simulink library "Pipe_Isolation"  (Simulink 8.2)
settings: Solver=ode45  StartTime=0.0  StopTime=10.0  RelTol=1e-3
libraries: carnot x4
settings Model: Creator=lena.frank  LastModifiedBy=drhf

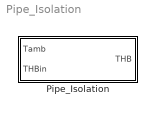
== system Pipe_Isolation ==
  Pipe_Isolation : Subsystem  mask(pipe with relative isolation thickness){dia=0.02, len=10, hgt=0, isolat=43.72, condiso=0.05, cond=0, cwall=1000, t0=20, lin=100/0.2, qua=100/0.2^2, nodes=10}
      mask prompts: dia "Diameter [m]"; len "Length of pipe [m]"; hgt "difference in static height [m], positive for outlet above"; isolat "Isolation thickness in % (100%: isolation thickness = diameter, minimum 1%)"; condiso "Thermal conductivity of isolation [W/(m*K)]"; cond "Effective conductivity in the pipe [W/(m*K)]"; cwall "capacity of pipewall per length in [J/(m*K)]"; t0 "initial temperature [degree centigrade]"; lin "pressure drop linear in massflow [Pa*s/kg]"; qua "pressure drop quadratic in massflow [Pa*s²/kg²]"; nodes "number of nodes"
      mask help:
      | Multinode pipe with capacity and easy pressure drop calculation. The pressure drop is a quadratic function of the massflow. The dependance of the quadratic term on the Reynolds number is neglected. The flow is calculated by the upwind scheme heat conduction between nodes by central differences (Patankar 1980).
      | Isolation thickness in percent of the diameter. Heat loss:
      | ul = 2*conductivity*pi*d*Length/Length/(d*log(((2*percent+1)d)/d))
      | The pressure change due to static height can usually be neglected for closes loop pumped systems.
      mask init:
      | if dia < 0.001
      |     dia = 0.001;
      |     disp('Warning in Pipe: diameter set to minimum value 0.001 m')
      | end
      | if len < 0.001
      |     len = 0.001;
      |     disp('Warning in Pipe: length set to minimum value 0.001 m')
      | end
      | if cwall < 0.001
      |     cwall = 0.001;
      |     disp('Warning in Pipe: heat capacity of the wall set to minimum value 0.001 m')
      | end
      | if nodes < 1
      |     nodes = 1;
      |     disp('Warning in Pipe: number of nodes set to minimum 1')
      | end
      | if isolat < 1
      |     isolat = 1;
      |     disp('Warning in Pipe: Isolation set to minimum 1%')
      | end
      | uloss = 2*condiso*pi/(log(0.01*isolat*2+1));
      mask Help: web(fullfile(path_carnot('help'),'Pipe_Isolation.html'),'-helpbrowser')
      mask Display: plot(-20,10,130,90,[0,2,5,7,5,2,0],[55,50,50,55,60,60,55],[96,99,100,99,96],[50,50,55,60,60],[10,13,17,19,19,17,13,10],[50,45,45,50,60,65,65,60],[5,15,17,17,15,5],[50,50,52,58,60,60],[17,93,96,96,92,17],[45,45,46,62,65,65])

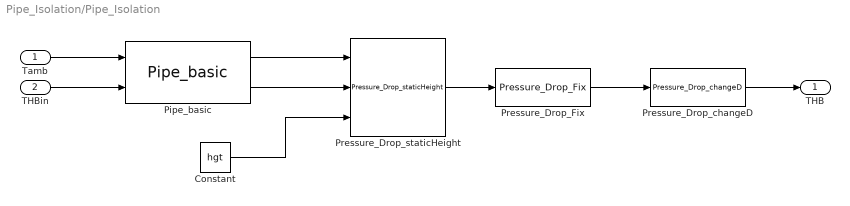
== system Pipe_Isolation/Pipe_Isolation ==
  Tamb : Inport
  THBin : Inport  Port=2
  Constant : Constant  Value=hgt
  Pipe_basic : carnot/Basic/Thermal_Models/Pipe_basic  vol=pi*(dia/2)^2*len  L=len  uloss=uloss  effcond=cond  cwall=cwall  t0=t0  nodes=nodes
  Pressure_Drop_Fix : carnot/Basic/Pressure_Drop/Pressure_Drop_Fix  con=0  lin=lin  qua=qua
  Pressure_Drop_changeD : carnot/Basic/Pressure_Drop/Pressure_Drop_changeD  dia=dia
  Pressure_Drop_staticHeight : carnot/Basic/Pressure_Drop/Pressure_Drop_staticHeight
  THB : Outport
  wires:
  Tamb/1 -> Pipe_basic/1
  THBin/1 -> Pipe_basic/2
  Constant/1 -> Pressure_Drop_staticHeight/3
  Pressure_Drop_staticHeight/1 -> Pressure_Drop_Fix/1
  Pressure_Drop_Fix/1 -> Pressure_Drop_changeD/1
  Pressure_Drop_changeD/1 -> THB/1
  Pipe_basic/1 -> Pressure_Drop_staticHeight/1
  Pipe_basic/2 -> Pressure_Drop_staticHeight/2
